simulink model "linearizedUnicycleRobotVSUnicycleRobot"  (R2024b)
settings: Solver=FixedStepAuto  StartTime=0.0  StopTime=10  FixedStep=0.001  RelTol=1e-3
values from neighbouring files (symbols this model uses):
  A = [ k1*v*cos(theta) 0 -v*sin(theta) ... (first row only)    [SimRun.m]
  B = [v*cos(1.17) 0 ... (first row only)    [SimRun.m]
  C = [1 0 0 ... (first row only)    [SimRun.m]
  D = [0 0 ... (first row only)    [SimRun.m]
settings Model: Creator=elija  LastModifiedBy=elija

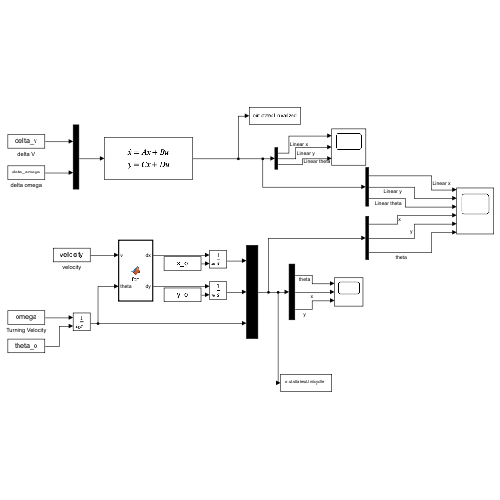
[thumbnail: Simulink's stored preview of the top-level diagram]
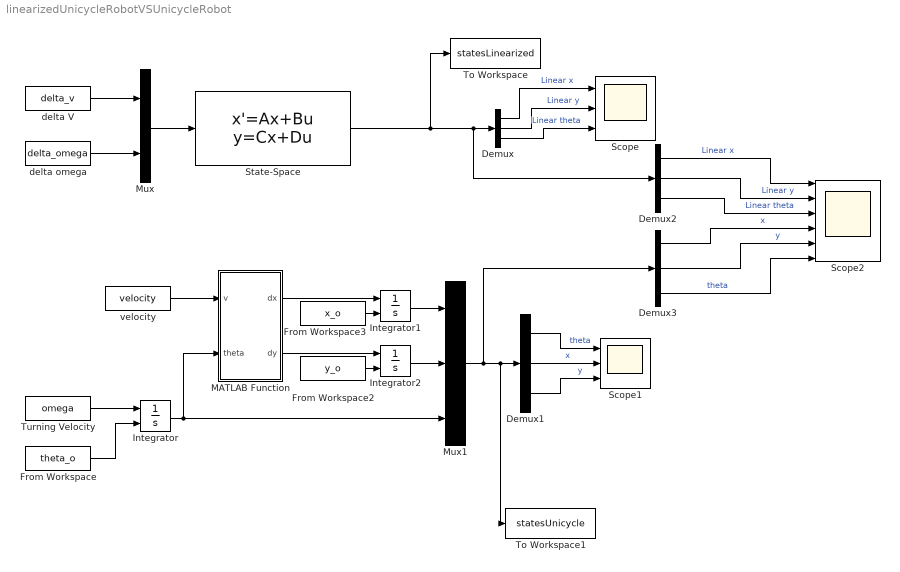
== system linearizedUnicycleRobotVSUnicycleRobot ==
  Demux{,1..3} (4 alike) : Demux  Outputs=3
  From Workspace : FromWorkspace  VariableName=theta_o
  From Workspace2 : FromWorkspace  VariableName=y_o
  From Workspace3 : FromWorkspace  VariableName=x_o
  Integrator : Integrator  InitialConditionSource=external
  Integrator1 : Integrator  InitialConditionSource=external
  Integrator2 : Integrator  InitialConditionSource=external
  MATLAB Function : MATLAB Function  TreatAsAtomicUnit=on
  Mux : Mux  Inputs=2
  Mux1 : Mux  Inputs=3
  Scope : Scope  NumInputPorts=3
  Scope1 : Scope  NumInputPorts=3
  Scope2 : Scope  NumInputPorts=6
  State-Space : StateSpace  A=A  B=B  C=C  D=D  InitialCondition=0
  To Workspace : ToWorkspace  VariableName=statesLinearized  SaveFormat=Timeseries  SampleTime=-1
  To Workspace1 : ToWorkspace  VariableName=statesUnicycle  SaveFormat=Timeseries  SampleTime=-1
  Turning Velocity : FromWorkspace  VariableName=omega
  delta V : FromWorkspace  VariableName=delta_v
  delta omega : FromWorkspace  VariableName=delta_omega
  velocity : FromWorkspace  VariableName=velocity
  wires:
  delta omega/1 -> Mux/2
  Mux/1 -> State-Space/1
  Demux/1 -> Scope/1  "Linear x"
  delta V/1 -> Mux/1
  Demux/2 -> Scope/2  "Linear y"
  Demux/3 -> Scope/3  "Linear theta"
  Mux1/1 -> Demux3/1, Demux1/1, To Workspace1/1
  velocity/1 -> MATLAB Function/1(v)
  From Workspace2/1 -> Integrator2/2
  Integrator/1 -> Mux1/3, MATLAB Function/2(theta)
  Integrator1/1 -> Mux1/1
  From Workspace3/1 -> Integrator1/2
  From Workspace/1 -> Integrator/2
  Turning Velocity/1 -> Integrator/1
  Integrator2/1 -> Mux1/2
  MATLAB Function/1(dx) -> Integrator1/1
  MATLAB Function/2(dy) -> Integrator2/1
  Demux1/1 -> Scope1/1  "theta"
  Demux1/2 -> Scope1/2  "x"
  Demux1/3 -> Scope1/3  "y"
  Demux2/2 -> Scope2/2  "Linear y"
  Demux2/1 -> Scope2/1  "Linear x"
  Demux2/3 -> Scope2/3  "Linear theta"
  Demux3/2 -> Scope2/5  "y"
  Demux3/3 -> Scope2/6  "theta"
  Demux3/1 -> Scope2/4  "x"
  State-Space/1 -> To Workspace/1, Demux2/1, Demux/1

== matlab function linearizedUnicycleRobotVSUnicycleRobot/MATLAB Function ==
  data: dx output; dy output; v input; theta input
function [dx,dy] = fcn(v,theta)

dx = v.*cos(theta);
dy = v.*sin(theta);


end
